simulink model "HeightModel_pid"  (R2018b)
settings: Solver=ode45  StartTime=0.0  StopTime=t_final  FixedStep=time_step  RelTol=1e-3
values from neighbouring files (symbols this model uses):
  bias_acc = 0    [mesh_generation.m]    (also in mesh_generation_normalized.m)
  gain = gain_grid(i)    [main.m]    (also in main_normalized.m = final_points_normalized(1,5); mesh_generation.m = gain_mesh(i2_gain); mesh_generation_normalized.m = 1)
  init_val = 0    [main.m]    (also in main_normalized.m = 0.001; mesh_generation.m; mesh_generation_normalized.m)
  Kd = x(2)    [get_step_cost_identified.m]    (also in mesh_generation.m = K(2); mesh_generation_normalized.m = K(2))
  Kp = x(1)    [get_step_cost_identified.m]    (also in mesh_generation.m = K(1); mesh_generation_normalized.m = K(1))
  ref_val = 1    [main.m]    (also in main_normalized.m = 0; mesh_generation.m; mesh_generation_normalized.m)
  sigma_h = 0*0.0005^2    (= 0)    [main.m]    (also in main_normalized.m = amplitude*0.05; mesh_generation.m; mesh_generation_normalized.m)
  T_body = T_body_grid(i)    [main.m]    (also in main_normalized.m = 0.2; mesh_generation.m = T_body_mesh(i2_T_body); mesh_generation_normalized.m = T_body_mesh(i2_T_body))
  T_prop = T_prop_grid(i)    [main.m]    (also in main_normalized.m = 0.015; mesh_generation.m = T_prop_mesh(i2_T_prop); mesh_generation_normalized.m = T_prop_mesh(i2_T_prop))
  tau = tau_grid(i)    [main.m]    (also in main_normalized.m = (0.1-0.001) * rand + 0.001; mesh_generation.m = tau_mesh(i2_tau); mesh_generation_normalized.m = tau_mesh(i2_tau))
  time_step = 0.0001    [main.m]    (also in main_normalized.m; mesh_generation.m = min([0.5*tau, 0.1*min([T_body, T_prop])]); mesh_generation_normalized.m = min([tau, 0.1*min([T_body, T_prop])]))
libraries: simulink x1
settings Model: Creator=mchehadeh  LastModifiedBy=aaa_b
settings DataIOCC: LimitDataPoints=on  SaveFormat=Array
settings OptimizationCC: BlockReduction=off  BooleanDataType=off  ExpressionDepthLimit=2147483647  LifeSpan=inf
settings DebuggingCC: SaveWithParameterizedLinksMsg=none  UnderspecifiedInitializationDetection=Classic  MergeDetectMultiDrivingBlocksExec=none  SignalResolutionControl=TryResolveAllWithWarning  MultiTaskDSMMsg=warning  MultiTaskCondExecSysMsg=none  StateNameClashWarn=warning  SFUnexpectedBacktrackingDiag=warning  SFNoUnconditionalDefaultTransitionDiag=warning  SFExecutionAtInitializationDiag=none
settings HardwareCC: ProdBitPerPointer=32  ProdBitPerSizeT=32  ProdBitPerPtrDiffT=32  ProdLargestAtomicFloat=None  ProdIntDivRoundTo=Undefined  ProdEndianess=Unspecified  ProdWordSize=32  ProdHWDeviceType=32-bit Generic  TargetUnknown=on
settings ModelReferenceCC: PropagateSignalLabelsOutOfModel=off
settings SFSimCC: SimUseLocalCustomCode=off
settings RTWCC: RTWUseLocalCustomCode=off
settings CodeAppCC: StateflowObjectComments=on
settings GRTTargetCC: TargetLangStandard=C89/C90 (ANSI)  GeneratePreprocessorConditionals=Disable all
settings ConfigComp: CovMetricSettings=dw  CovHtmlReporting=on  CovSaveCumulativeToWorkspaceVar=on  CovSaveSingleToWorkspaceVar=on  CovExternalEMLEnable=off

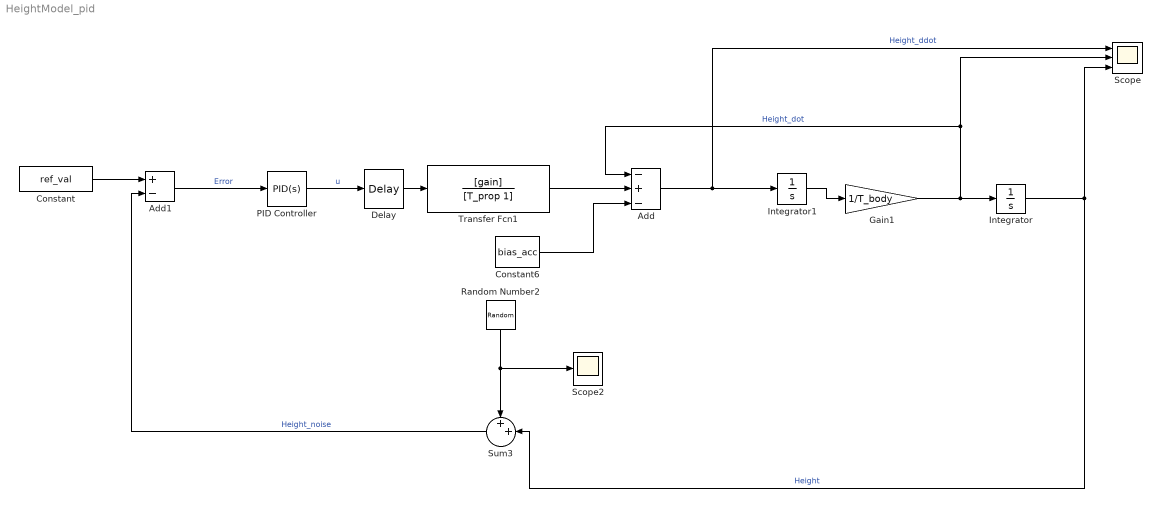
== system HeightModel_pid ==
  Add : Sum  Inputs=-+-
  Add1 : Sum  Inputs=+-
  Constant : Constant  Value=ref_val
  Constant6 : Constant  Value=bias_acc
  "Delay " : TransportDelay  DelayTime=tau  InitialOutput=init_val
  Gain1 : Gain  Gain=1/T_body
  Integrator : Integrator  InitialCondition=init_val  LimitOutput=on  LowerSaturationLimit=0
  Integrator1 : Integrator
  PID Controller : simulink/Continuous/PID Controller  Controller=PID  Form=Parallel  TimeDomain=Continuous-time  SampleTime=1  IntegratorMethod=Forward Euler  FilterMethod=Forward Euler  ControllerParametersSource=internal  P=Kp  I=Kd  D=0  UseFilter=on  N=1e6  TunerSelectOption=Transfer Function Based (PID Tuner App)  InitialConditionSource=internal  InitialConditionForIntegrator=0  InitialConditionForFilter=0  DifferentiatorICPrevScaledInput=0  ExternalReset=none  TrackingMode=off  Kt=1  LimitOutput=off  UpperSaturationLimit=inf  LowerSaturationLimit=-inf  LinearizeAsGain=on  AntiWindupMode=none  Kb=1  POutMin=[]  POutMax=[]  IOutMin=[]  IOutMax=[]  DOutMin=[]  DOutMax=[]  NOutMin=[]  NOutMax=[]  SumOutMin=[]  SumOutMax=[]  SaturationOutMin=[]  SaturationOutMax=[]  PParamMin=[]  PParamMax=[]  IParamMin=[]  IParamMax=[]  DParamMin=[]  DParamMax=[]  NParamMin=[]  NParamMax=[]  KbParamMin=[]  KbParamMax=[]  KtParamMin=[]  KtParamMax=[]  KbOutMin=[]  KbOutMax=[]  KtOutMin=[]  KtOutMax=[]  IntegratorOutMin=[]  IntegratorOutMax=[]  FilterOutMin=[]  FilterOutMax=[]  SumI1OutMin=[]  SumI1OutMax=[]  SumI2OutMin=[]  SumI2OutMax=[]  SumI3OutMin=[]  SumI3OutMax=[]  SumI4OutMin=[]  SumI4OutMax=[]  SumDOutMin=[]  SumDOutMax=[]  DifferentiatorOutMin=[]  DifferentiatorOutMax=[]  FilterDiffOutCoefMin=[]  FilterDiffOutCoefMax=[]  ReciprocalOutMin=[]  ReciprocalOutMax=[]  SumDenOutMin=[]  SumDenOutMax=[]  SumNumOutMin=[]  SumNumOutMax=[]  DivideOutMin=[]  DivideOutMax=[]  IntegratorContinuousStateAttributes=''  IntegratorStateMustResolveToSignalObject=off  IntegratorRTWStateStorageClass=Auto  FilterContinuousStateAttributes=''  FilterStateMustResolveToSignalObject=off  FilterRTWStateStorageClass=Auto  ParallelPVariant=InternalParameters  IdealPVariant=Disabled  IVariant=InternalParameters  DVariant=InternalParameters  IntegratorVariant=Continuous  SatVariant=Disabled  AWVariant=Passthrough  PCopyVariant=Disabled  TRVariant=Disabled  FdbkBlocksVariant=Forward  IdealPFdbkVariant=Disabled  SatFdbkVariant=Disabled  DerivativeFilterVariant=ContFilter  NVariant=InternalParameters  NCopyVariant=Disabled  FilterICVariant=InternalICsFilter  IntegratorICVariant=InternalICs  ExternalResetVariant=Disabled  TRSumVariant=Passthrough  SumFdbkVariant=Disabled  SumVariant=Sum_PID
  Random Number2 : RandomNumber  Variance=sigma_h  SampleTime=time_step
  Scope : Scope  NumInputPorts=3
  Scope2 : Scope
  Sum3 : Sum  Inputs=++|
  Transfer Fcn1 : TransferFcn  Numerator=[gain]  Denominator=[T_prop 1]
  wires:
  Gain1/1 -> Scope/2, Add/1, Integrator/1  "Height_dot"
  Integrator/1 -> Scope/3, Sum3/2  "Height"
  Constant/1 -> Add1/1
  Sum3/1 -> Add1/2  "Height_noise"
  Random Number2/1 -> Scope2/1, Sum3/1
  Add/1 -> Scope/1, Integrator1/1  "Height_ddot"
  Constant6/1 -> Add/3
  "Delay "/1 -> Transfer Fcn1/1
  Transfer Fcn1/1 -> Add/2
  Integrator1/1 -> Gain1/1
  PID Controller/1 -> "Delay "/1  "u"
  Add1/1 -> PID Controller/1  "Error"
